simulink model "SS_jun_25"  (R2014b)
settings: Solver=ode45  StartTime=0.0  StopTime=50.0  RelTol=1e-3
libraries: simulink x1
settings Model: Creator=Bismaya  LastModifiedBy=Bismaya

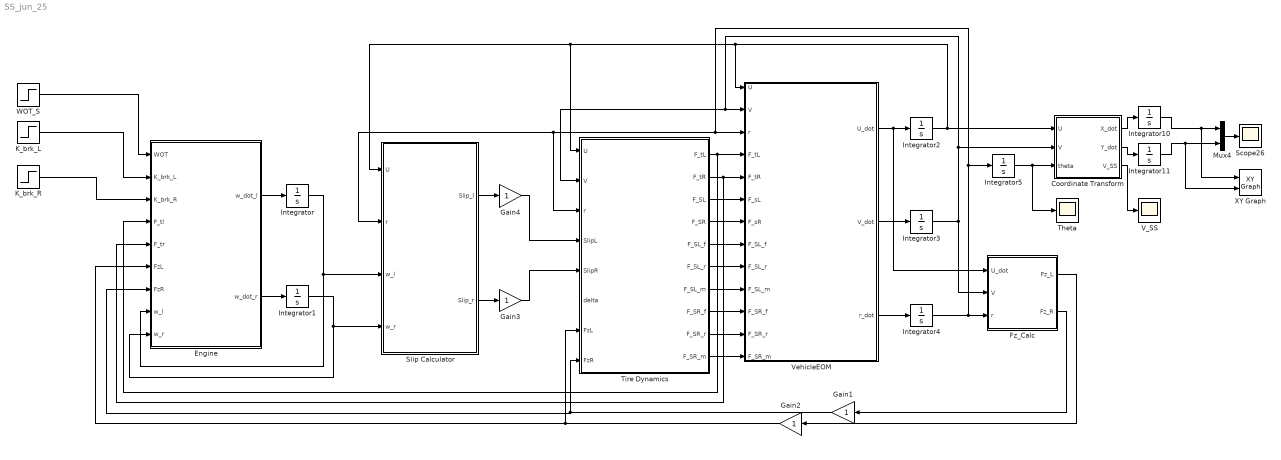
== system SS_jun_25 ==
  Coordinate Transform : MATLAB Function  TreatAsAtomicUnit=on
  Engine : MATLAB Function  TreatAsAtomicUnit=on
  Fz_Calc : MATLAB Function  TreatAsAtomicUnit=on
  Gain{1..4} (4 alike) : Gain
  Integrator : Integrator  InitialCondition=12  LowerSaturationLimit=-0.0001
  Integrator1 : Integrator  InitialCondition=12  LowerSaturationLimit=-0.0001
  Integrator{3..5,10..11} (5 alike) : Integrator
  Integrator2 : Integrator  InitialCondition=10/3
  K_brk_L : Step  Time=0  After=0  SampleTime=0
  K_brk_R : Step  Time=20  After=40  SampleTime=0
  Mux4 : Mux  Inputs=2
  Scope26 : Scope
      settings: YMin=-50  YMax=200  SaveName=XY
  Slip Calculator : MATLAB Function  TreatAsAtomicUnit=on
  Theta : Scope
      settings: YMin=20  YMax=45  SaveName=Theta
  Tire Dynamics : Subsystem
  V_SS : Scope
      settings: YMin=20  YMax=45  SaveName=Theta1
  VehicleEOM : MATLAB Function  TreatAsAtomicUnit=on
  "WOT_S " : Step  Time=0  Before=1  SampleTime=0
  XY Graph : simulink/Sinks/XY Graph  xmin=-250  xmax=250  ymin=-250  ymax=250  st=-1
  wires:
  Engine/1(w_dot_l) -> Integrator/1
  Engine/2(w_dot_r) -> Integrator1/1
  Integrator1/1 -> Engine/9(w_r), Slip Calculator/4(w_r)
  Slip Calculator/1(Slip_l) -> Gain4/1
  Slip Calculator/2(Slip_r) -> Gain3/1
  Integrator/1 -> Slip Calculator/3(w_l), Engine/8(w_l)
  "WOT_S "/1 -> Engine/1(WOT)
  Tire Dynamics/10(F_SR_m) -> VehicleEOM/13(F_SR_m)
  Tire Dynamics/9(F_SR_r) -> VehicleEOM/12(F_SR_r)
  Tire Dynamics/8(F_SR_f) -> VehicleEOM/11(F_SR_f)
  Tire Dynamics/7(F_SL_m) -> VehicleEOM/10(F_SL_m)
  Tire Dynamics/6(F_SL_r) -> VehicleEOM/9(F_SL_r)
  Tire Dynamics/5(F_SL_f) -> VehicleEOM/8(F_SL_f)
  Tire Dynamics/4(F_SR) -> VehicleEOM/7(F_sR)
  Tire Dynamics/3(F_SL) -> VehicleEOM/6(F_sL)
  Tire Dynamics/2(F_tR) -> Engine/5(F_tr), VehicleEOM/5(F_tR)
  Tire Dynamics/1(F_tL) -> Engine/4(F_tl), VehicleEOM/4(F_tL)
  K_brk_L/1 -> Engine/2(K_brk_L)
  K_brk_R/1 -> Engine/3(K_brk_R)
  VehicleEOM/1(U_dot) -> Fz_Calc/1(U_dot), Integrator2/1
  VehicleEOM/2(V_dot) -> Integrator3/1
  VehicleEOM/3(r_dot) -> Integrator4/1
  Integrator2/1 -> Tire Dynamics/1(U), Slip Calculator/1(U), VehicleEOM/1(U), Coordinate Transform/1(U)
  Integrator3/1 -> Tire Dynamics/2(V), VehicleEOM/2(V), Coordinate Transform/2(V), Fz_Calc/2(V)
  Integrator4/1 -> Tire Dynamics/3(r), Slip Calculator/2(r), VehicleEOM/3(r), Integrator5/1, Fz_Calc/3(r)
  Fz_Calc/2(Fz_R) -> Gain1/1
  Fz_Calc/1(Fz_L) -> Gain2/1
  Integrator5/1 -> Coordinate Transform/3(theta), Theta/1
  Coordinate Transform/1(X_dot) -> Integrator10/1
  Coordinate Transform/2(Y_dot) -> Integrator11/1
  Integrator11/1 -> XY Graph/2, Mux4/2
  Integrator10/1 -> XY Graph/1, Mux4/1
  Mux4/1 -> Scope26/1
  Coordinate Transform/3(V_SS) -> V_SS/1
  Gain1/1 -> Engine/7(FzR), Tire Dynamics/8(FzR)
  Gain2/1 -> Engine/6(FzL), Tire Dynamics/7(FzL)
  Gain3/1 -> Tire Dynamics/5(SlipR)
  Gain4/1 -> Tire Dynamics/4(SlipL)

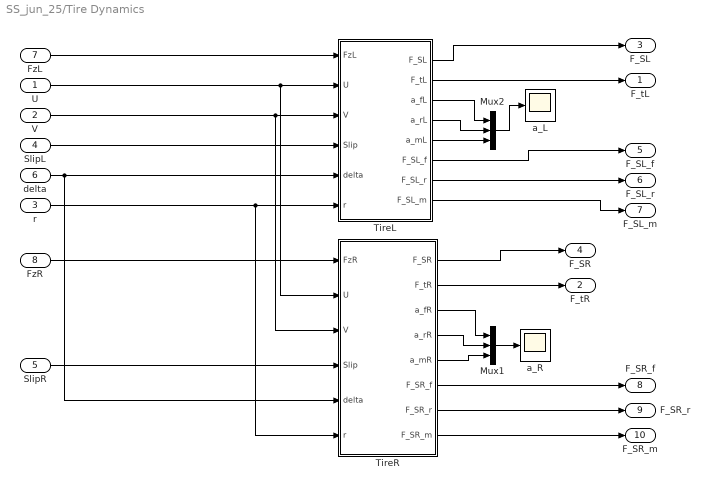
== system SS_jun_25/Tire Dynamics ==
  U : Inport
  V : Inport  Port=2
  r : Inport  Port=3
  SlipL : Inport  Port=4
  SlipR : Inport  Port=5
  delta : Inport  Port=6
  FzL : Inport  Port=7
  FzR : Inport  Port=8
  Mux1 : Mux  Inputs=3
  Mux2 : Mux  Inputs=3
  TireL : MATLAB Function  TreatAsAtomicUnit=on
  TireR : MATLAB Function  TreatAsAtomicUnit=on
  a_L : Scope
      settings: YMin=20  YMax=45  SaveName=a_L  MaxDataPoints=5000000
  a_R : Scope
      settings: YMin=20  YMax=45  SaveName=a_R  MaxDataPoints=5000000
  F_tL : Outport
  F_tR : Outport  Port=2
  F_SL : Outport  Port=3
  F_SR : Outport  Port=4
  F_SL_f : Outport  Port=5
  F_SL_r : Outport  Port=6
  F_SL_m : Outport  Port=7
  F_SR_f : Outport  Port=8
  F_SR_r : Outport  Port=9
  F_SR_m : Outport  Port=10
  wires:
  TireL/8(F_SL_m) -> F_SL_m/1
  U/1 -> TireL/2(U), TireR/2(U)
  FzR/1 -> TireR/1(FzR)
  delta/1 -> TireR/5(delta), TireL/5(delta)
  SlipR/1 -> TireR/4(Slip)
  V/1 -> TireR/3(V), TireL/3(V)
  TireR/1(F_SR) -> F_SR/1
  r/1 -> TireR/6(r), TireL/6(r)
  TireL/2(F_tL) -> F_tL/1
  TireL/6(F_SL_f) -> F_SL_f/1
  SlipL/1 -> TireL/4(Slip)
  TireL/7(F_SL_r) -> F_SL_r/1
  FzL/1 -> TireL/1(FzL)
  TireL/1(F_SL) -> F_SL/1
  Mux2/1 -> a_L/1
  TireR/3(a_fR) -> Mux1/1
  TireR/4(a_rR) -> Mux1/2
  Mux1/1 -> a_R/1
  TireR/5(a_mR) -> Mux1/3
  TireR/2(F_tR) -> F_tR/1
  TireR/6(F_SR_f) -> F_SR_f/1
  TireR/7(F_SR_r) -> F_SR_r/1
  TireR/8(F_SR_m) -> F_SR_m/1
  TireL/5(a_mL) -> Mux2/3
  TireL/3(a_fL) -> Mux2/1
  TireL/4(a_rL) -> Mux2/2

== matlab function SS_jun_25/Engine ==
  data: WOT input; K_brk_L input; K_brk_R input; F_tl input; F_tr input; FzL input; FzR input; w_l input; w_r input; w_dot_l output; w_dot_r output
function [w_dot_l,w_dot_r] = engine_model(WOT,K_brk_L,K_brk_R,F_tl,F_tr,FzL,FzR,w_l,w_r)
M=1280;Ms=1160;Izz=2500;Ixx=750;Ixz=0;a=1.203;b=1.217;hcg=0.5;e=0.2;Tw=1.33;R=0.3;I_t=2.1;
I_e=0.136;A_f=2.1;zi1=2.5*13.56;zi2=7.50;zi3=5.37;zi4=4.22;zi5=3.28;
Lbpsi=45000;Lbp=2600;C_a=20000;C_i=20000;mu=0.85;e_r=0.015;K_rsf=-0.05;K_rsr=0.1;
C1=-6.0;C2=59.16;C3=25;C_s1=1.38;K_rsf=0.444;C_d=0.32;d=0.014;n=0.85;
rho=1.204;g=9.81;
K_bf=0.55;
zi=zi1*2;

F_tl=F_tl;
F_tr=F_tr;
F_t1=F_tl+F_tr;
%Engine Equations
w_el=zi*w_l;
w_er=zi*w_r;

IwL=I_t+(0.5*zi*zi*n*I_e);%Accelerating
IwR=I_t+(0.5*zi*zi*n*I_e);%Accelerating

T_l=WOT*zi*n*(C1*(w_el/100)^2+C2*(w_el/100)+C3);
T_r=WOT*zi*n*(C1*(w_er/100)^2+C2*(w_er/100)+C3);
T_trac_L=T_l-(R*F_tl)-(d*FzL);
T_trac_R=T_r-(R*F_tr)-(d*FzR);
T_brkl=K_brk_L*T_l;
T_brkr=K_brk_R*T_r;
w_dot_l=(1/(IwL))*(T_trac_L-T_brkl);
w_dot_r=(1/(IwR))*(T_trac_R-T_brkr);
% w_dot_f=(1/Iw)*(T_f-(d*Fzf)-(0.5*T_brkf));
% w_dot_r=(1/Iw)*(T_r-(d*Fzr)-(0.5*T_brkr));

== matlab function SS_jun_25/Tire Dynamics/TireR ==
  data: FzR input; F_SR output; F_tR output; U input; V input; Slip input; delta input; r input; a_fR output; a_rR output; a_mR output; F_SR_f output; F_SR_r output; F_SR_m output
function [F_SR,F_tR,a_fR,a_rR,a_mR,F_SR_f,F_SR_r,F_SR_m] = tireR(FzR,U,V,Slip,delta,r)
M=1280;Ms=1160;Izz=2500;Ixx=750;Ixz=0;a=1.203;b=1.217;hcg=0.5;e=0.2;Tw=1.33;R=0.3;I_t=2.1;
I_e=0.136;A_f=2.1;K_bf=0.55;zi1=13.56;z2=7.50;zi3=5.37;zi4=4.22;zi5=3.28;
Lbpsi=45000;Lbp=2600;C_a=20000;C_i=20000;mu=0.85;e_r=0.015;K_rsf=-0.05;K_rsr=0.1;
C1=-6.0;C2=59.16;C3=25;C_s1=1.38;K_rsf=0.444;C_d=0.32;d=0.014;n=0.85;
rho=1.204;g=9.81;c=0.2;


% FzF=M*g*mu/2;
Fz=FzR;

%Tire Longitudinal Velocity Calculation
% U_tf=U*cos(delta)+(V+a*r)*sin(delta);
% U_tr=U;

 %Side Slip Calc
a_fR=-atan((V+a*r)/(U-0.5*Tw*r));
a_rR=atan((b*r-V)/(U-0.5*Tw*r));
a_mR=atan((c*r-V)/(U-0.5*Tw*r));

alpha=a_fR;

 U_tl=U+(0.5*Tw*r);
 U_tr=U-(0.5*Tw*r);
%%FRONT Tires
%Tire Equations
S_f=(mu*(Fz/3)*(1-(e_r*U_tr*sqrt((Slip*Slip)+(tan(alpha)*tan(alpha)))))*(1-Slip))/...
    (2*sqrt(C_i*C_i*Slip*Slip+C_a*C_a*tan(alpha)*tan(alpha)));
if(S_f<1)
    f_S=S_f*(2-S_f);
else
    f_S=1;
end
F_SR_f=(C_a*tan(alpha)*f_S)/(1-Slip);
F_tR_f=(C_i*Slip*f_S)/(1-Slip);

%%Rear Tires
alpha=a_rR;

S_r=(mu*(Fz/3)*(1-(e_r*U_tr*sqrt((Slip*Slip)+(tan(alpha)*tan(alpha)))))*(1-Slip))/...
    (2*sqrt(C_i*C_i*Slip*Slip+C_a*C_a*tan(alpha)*tan(alpha)));
if(S_r<1)
    f_S=S_r*(2-S_r);
else
    f_S=1;
end
F_SR_r=(C_a*tan(alpha)*f_S)/(1-Slip);
F_tR_r=(C_i*Slip*f_S)/(1-Slip);

%%Middle Tires
alpha=a_mR;

S_m=(mu*(Fz/3)*(1-(e_r*U_tr*sqrt((Slip*Slip)+(tan(alpha)*tan(alpha)))))*(1-Slip))/...
    (2*sqrt(C_i*C_i*Slip*Slip+C_a*C_a*tan(alpha)*tan(alpha)));
if(S_m<1)
    f_S=S_m*(2-S_m);
else
    f_S=1;
end
F_SR_m=(C_a*tan(alpha)*f_S)/(1-Slip);
F_tR_m=(C_i*Slip*f_S)/(1-Slip);


F_SR=F_SR_f+F_SR_r+F_SR_m;
F_tR=F_tR_f+F_tR_r+F_tR_m;
F_R=[F_tR_f;F_tR_r;F_tR_m;F_SR_f;F_SR_r;F_SR_m];

== matlab function SS_jun_25/VehicleEOM ==
  data: U input; V input; U_dot output; V_dot output; r input; F_tL input; F_tR input; F_sL input; F_sR input; r_dot output; F_SL_f input; F_SL_r input; F_SL_m input; F_SR_f input; F_SR_r input; F_SR_m input
function [U_dot,V_dot,r_dot] = VehicleEOM(U,V,r,F_tL,F_tR,F_sL,F_sR,F_SL_f,F_SL_r,F_SL_m,F_SR_f,F_SR_r,F_SR_m)
M=1280;Ms=1160;Izz=2500;Ixx=750;Ixz=0;a=1.203;b=1.217;hcg=0.5;e=0.2;Tw=1.33;R=0.3;I_t=2.1;
I_e=0.136;A_f=2.1;K_bf=0.55;zi1=13.56;z2=7.50;zi3=5.37;zi4=4.22;zi5=3.28;
Lbpsi=45000;Lbp=2600;C_a=20000;C_i=20000;mu=0.85;e_r=0.015;K_rsf=-0.05;K_rsr=0.1;
C1=-6.0;C2=59.16;C3=25;C_s1=1.38;K_rsf=0.444;C_d=0.32;d=0.014;n=0.85;
rho=1.204;g=9.81;c=0.2;

F_t=(F_tL+F_tR);
%Vehicle Equations
% U_dot=(1/M)*((M*V*r)+F_t-(0.5*C_d*A_f*rho*U*U));
U_dot=(1/M)*((M*V*r)+F_t);

V_dot=(1/M)*((-M*U*r)+F_sL+F_sR);
% r_dot=(1/Izz)*(2*a*F_tL*sin(delta)+2*a*F_sL*cos(delta)-2*b*F_sR);
 r_dot=(1/(0.5*Izz))*(0.5*Tw*F_tL-0.5*Tw*F_tR+a*(F_SL_f+F_SR_f)-b*(F_SL_r+F_SR_r)-c*(F_SL_m+F_SR_m));

== matlab function SS_jun_25/Slip Calculator ==
  data: U input; r input; w_l input; w_r input; Slip_l output; Slip_r output
function [Slip_l,Slip_r] = slipCalculator(U,r,w_l,w_r)
M=1280;Ms=1160;Izz=2500;Ixx=750;Ixz=0;a=1.203;b=1.217;hcg=0.5;e=0.2;Tw=1.33;R=0.3;I_t=2.1;
I_e=0.136;A_f=2.1;K_bf=0.55;zi1=13.56;z2=7.50;zi3=5.37;zi4=4.22;zi5=3.28;
Lbpsi=45000;Lbp=2600;C_a=20000;C_i=20000;mu=0.85;e_r=0.015;K_rsf=-0.05;K_rsr=0.1;
C1=-6.0;C2=59.16;C3=25;C_s1=1.38;K_rsf=0.444;C_d=0.32;d=0.014;n=0.85;
rho=1.204;g=9.81;

% w_r=-w_r;
% w_f=-w_f;
%Tire Longitudinal Velocity Calculation
% U_tl=U*cos(delta)+(V+a*r)*sin(delta);
% U_tr=U;
 U_tl=U+(0.5*Tw*r);
 U_tr=U-(0.5*Tw*r);

% %  SlipCalc
% if(U_tl<=(R*w_l))
%     Slip_l=1-(U_tl/(R*w_l));%Acceleration
% else
%     Slip_l=1-((R*w_l)/U_tl);%Braking
% %     Slip_l=0;
% end
% 
% if(U_tr<=(R*w_r))
%     Slip_r=1-(U_tr/(R*w_r));%Acceleration
% else
%     Slip_r=1-((R*w_r)/U_tr);%Braking
% %     Slip_r=0;
% end
Slip_l=1-(U_tl/(R*w_l));
Slip_r=1-(U_tr/(R*w_r));

% 
% if(Slip_l<0)
%      Slip_l=0;
%  elseif (Slip_l>1)
%          Slip_l=1;
%  end
%  if(Slip_r<0)
%      Slip_r=0;
%  elseif (Slip_r>1)
%          Slip_r=1;
%  end
% %

== matlab function SS_jun_25/Fz_Calc ==
  data: U_dot input; V input; Fz_L output; Fz_R output; r input
function [Fz_L,Fz_R] = FzCalc(U_dot,V,r)
M=1280;Ms=1160;Izz=2500;Ixx=750;Ixz=0;a=1.203;b=1.217;hcg=0.5;e=0.2;Tw=1.33;R=0.3;I_t=2.1;
I_e=0.136;A_f=2.1;K_bf=0.55;zi1=13.56;z2=7.50;zi3=5.37;zi4=4.22;zi5=3.28;
Lbpsi=45000;Lbp=2600;C_a=20000;C_i=20000;mu=0.85;e_r=0.015;K_rsf=-0.05;K_rsr=0.1;
C1=-6.0;C2=59.16;C3=25;C_s1=1.38;K_rsf=0.444;C_d=0.32;d=0.014;n=0.85;
rho=1.204;g=9.81;


%NormalForceCalc
% Fz_f=(M*g/2)*((b/(a+b))-((U_dot-V*r)*hcg)/(g*(a+b)));
% Fz_r=(M*g/2)*((a/(a+b))+((U_dot-V*r)*hcg)/(g*(a+b)));
Fz_L=(M*g/2);
Fz_R=(M*g/2);

== matlab function SS_jun_25/Tire Dynamics/TireL ==
  data: FzL input; F_SL output; F_tL output; U input; V input; Slip input; delta input; r input; a_fL output; a_rL output; a_mL output; F_SL_f output; F_SL_r output; F_SL_m output
function [F_SL,F_tL,a_fL,a_rL,a_mL,F_SL_f,F_SL_r,F_SL_m] = tireL(FzL,U,V,Slip,delta,r)
M=1280;Ms=1160;Izz=2500;Ixx=750;Ixz=0;a=1.203;b=1.217;hcg=0.5;e=0.2;Tw=1.33;R=0.3;I_t=2.1;
I_e=0.136;A_f=2.1;K_bf=0.55;zi1=13.56;z2=7.50;zi3=5.37;zi4=4.22;zi5=3.28;
Lbpsi=45000;Lbp=2600;C_a=20000;C_i=20000;mu=0.85;e_r=0.015;K_rsf=-0.05;K_rsr=0.1;
C1=-6.0;C2=59.16;C3=25;C_s1=1.38;K_rsf=0.444;C_d=0.32;d=0.014;n=0.85;
rho=1.204;g=9.81;c=0.2;


% FzF=M*g*mu/2;

Fz=FzL;

%Tire Longitudinal Velocity Calculation
% U_tf=U*cos(delta)+(V+a*r)*sin(delta);
% U_tr=U;
 U_tl=U+(0.5*Tw*r);
 U_tr=U-(0.5*Tw*r);
%FRONT Tires
 %Side Slip Calc
a_fL=-atan((V+a*r)/(U+0.5*Tw*r));
a_rL=atan((b*r-V)/(U+0.5*Tw*r));
a_mL=atan((c*r-V)/(U+0.5*Tw*r));

alpha=a_fL;
%Tire Equations
S_f=(mu*(Fz/3)*(1-(e_r*U_tl*sqrt((Slip*Slip)+(tan(alpha)*tan(alpha)))))*(1-Slip))/...
    (2*sqrt(C_i*C_i*Slip*Slip+C_a*C_a*tan(alpha)*tan(alpha)));
if(S_f<1)
    f_S=S_f*(2-S_f);
else
    f_S=1;
end
F_SL_f=(C_a*tan(alpha)*f_S)/(1-Slip);
F_tL_f=(C_i*Slip*f_S)/(1-Slip);

%Rear Tires
alpha=a_rL;

S_r=(mu*(Fz/3)*(1-(e_r*U_tl*sqrt((Slip*Slip)+(tan(alpha)*tan(alpha)))))*(1-Slip))/...
    (2*sqrt(C_i*C_i*Slip*Slip+C_a*C_a*tan(alpha)*tan(alpha)));
if(S_r<1)
    f_S=S_r*(2-S_r);
else
    f_S=1;
end
F_SL_r=(C_a*tan(alpha)*f_S)/(1-Slip);
F_tL_r=(C_i*Slip*f_S)/(1-Slip);

%Middle Tires
alpha=a_mL;

S_m=(mu*(Fz/3)*(1-(e_r*U_tl*sqrt((Slip*Slip)+(tan(alpha)*tan(alpha)))))*(1-Slip))/...
    (2*sqrt(C_i*C_i*Slip*Slip+C_a*C_a*tan(alpha)*tan(alpha)));
if(S_m<1)
    f_S=S_m*(2-S_m);
else
    f_S=1;
end
F_SL_m=(C_a*tan(alpha)*f_S)/(1-Slip);
F_tL_m=(C_i*Slip*f_S)/(1-Slip);


F_SL=F_SL_f+F_SL_r+F_SL_m;
F_tL=F_tL_f+F_tL_r+F_tL_m;
F_L=[F_tL_f;F_tL_r;F_tL_m;F_SL_f;F_SL_r;F_SL_m;];

== matlab function SS_jun_25/Coordinate Transform ==
  data: U input; V input; theta input; X_dot output; Y_dot output; V_SS output
function [X_dot,Y_dot, V_SS] = CT(U,V,theta)
M=1280;Ms=1160;Izz=2500;Ixx=750;Ixz=0;a=1.203;b=1.217;hcg=0.5;e=0.2;Tw=1.33;R=0.3;I_t=2.1;
I_e=0.136;A_f=2.1;K_bf=0.55;zi1=13.56;z2=7.50;zi3=5.37;zi4=4.22;zi5=3.28;
Lbpsi=45000;Lbp=2600;C_a=20000;C_i=20000;mu=0.85;e_r=0.015;K_rsf=-0.05;K_rsr=0.1;
C1=-6.0;C2=59.16;C3=25;C_s1=1.38;K_rsf=0.444;C_d=0.32;d=0.014;n=0.85;
rho=1.204;g=9.81;c=0.2;

% X_dot=U*cos(theta)-V*sin(theta);
% Y_dot=+U*sin(theta)+V*cos(theta);
X_dot=U*sin(theta)+V*cos(theta);
Y_dot=U*cos(theta)-V*sin(theta);
V_SS=atand(V/U);
